simulink model "case_10_lead_gradually_slows_down"  (R2025b)
settings: Solver=VariableStepAuto  StartTime=0.0  StopTime=20  RelTol=1e-3
settings Model: Creator=sanborkl  LastModifiedBy=admin

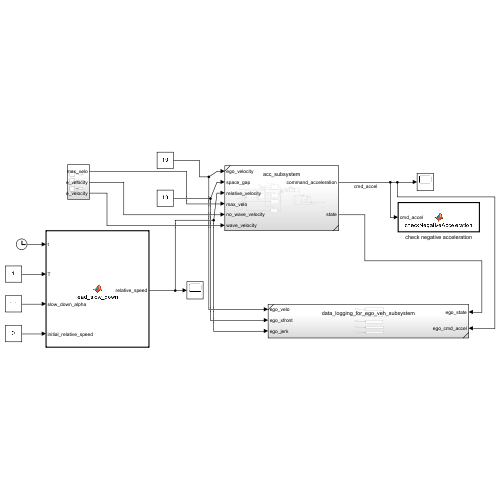
[thumbnail: Simulink's stored preview of the top-level diagram]
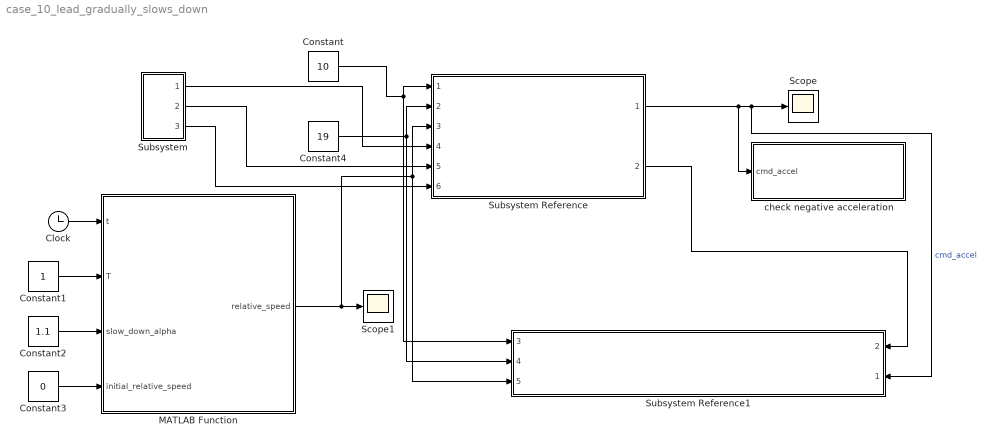
== system case_10_lead_gradually_slows_down ==
  Clock : Clock
  Constant : Constant  Value=10
  Constant1 : Constant
  Constant2 : Constant  Value=1.1
  Constant3 : Constant  Value=0
  Constant4 : Constant  Value=19
  MATLAB Function : MATLAB Function  TreatAsAtomicUnit=on
  Scope : Scope
      settings: ActiveDisplayYMinimum=-2.5  ActiveDisplayYMaximum=-0.5
  Scope1 : Scope
      settings: ActiveDisplayYMinimum=-20.642422203963303  ActiveDisplayYMaximum=8.4753069399564325
  Subsystem : Subsystem
  Subsystem Reference : Subsystem  ReferencedSubsystem=acc_subsystem
  Subsystem Reference1 : Subsystem  ReferencedSubsystem=data_logging_for_ego_veh_subsystem
      settings: PortSchema="{\"entries\":[{\"content\":{\"sides\":[{\"content\":{\"connectorIds\":[\"In3\",\"In4\",\"In5\"]},\"type\":\"ConnectorPlacement.EquallySpacedRectSide\",\"uuid\":\"0b96bcaa-a470-46c9-9268-f4bd6b1035a8\"},{\"content\":{\"connectorIds\":[\"In2\",\"In1\"],\"side\":\"RIGHT\"},\"type\":\"ConnectorPlacement.EquallySpacedRectSide\",\"uuid\":\"8e49005a-1e53-4e76-b163-50df0eb9f2cc\"},{\"content\":{\"side\":\"TOP\"},\"type\":\"ConnectorPlacement.EquallySpacedRectSide\",\"uuid\":\"3ff4af65-efca-4a64-9b7f-f479498e89e2\"}]},\"type\":\"ConnectorPlacement.EquallySpacedConnector\",\"uuid\":\"f10caef7-9599-4d5c-a8fd-3eb49f6fcaa8\"}],\"packageUris\":[\"http://schema.mathworks.com/mf0/Connector/R2020b\"],\"version\":\"1.0\"}"
  check negative acceleration : MATLAB Function  TreatAsAtomicUnit=on
  wires:
  Constant/1 -> Subsystem Reference1/3, Subsystem Reference/1
  Clock/1 -> MATLAB Function/1(t)
  Constant1/1 -> MATLAB Function/2(T)
  Constant2/1 -> MATLAB Function/3(slow_down_alpha)
  Constant3/1 -> MATLAB Function/4(initial_relative_speed)
  MATLAB Function/1(relative_speed) -> Subsystem Reference1/5, Subsystem Reference/3, Scope1/1
  Constant4/1 -> Subsystem Reference1/4, Subsystem Reference/2
  Subsystem Reference/1 -> check negative acceleration/1(cmd_accel), Subsystem Reference1/1, Scope/1  "cmd_accel"
  Subsystem Reference/2 -> Subsystem Reference1/2
  Subsystem/1(max_velo) -> Subsystem Reference/4
  Subsystem/2(no_wave_velocity) -> Subsystem Reference/5
  Subsystem/3(wave_velocity) -> Subsystem Reference/6

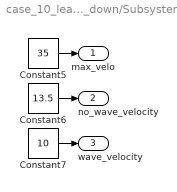
== system case_10_lead_gradually_slows_down/Subsystem ==
  Constant5 : Constant  Value=35
  Constant6 : Constant  Value=13.5
  Constant7 : Constant  Value=10
  max_velo : Outport
  no_wave_velocity : Outport  Port=2
  wave_velocity : Outport  Port=3
  wires:
  Constant7/1 -> wave_velocity/1
  Constant6/1 -> no_wave_velocity/1
  Constant5/1 -> max_velo/1

== matlab function case_10_lead_gradually_slows_down/MATLAB Function ==
  data: t input; relative_speed output; T input; slow_down_alpha input; initial_relative_speed input
function relative_speed = lead_slow_down(t, T, slow_down_alpha, initial_relative_speed)

if (t < T)
    relative_speed = initial_relative_speed;
else
    relative_speed = initial_relative_speed + -(slow_down_alpha * t);
end

== matlab function case_10_lead_gradually_slows_down/check negative acceleration ==
  data: cmd_accel input
function checkNegativeAcceleration(cmd_accel)
%#codegen
coder.extrinsic('disp', 'sprintf');

if cmd_accel > 0
    msg = sprintf('Error: Positive command acceleration: %.3f, should be negative', ...
                  cmd_accel);
    disp(msg);
end
end
